simulink model "LQR_lpfnoise"  (R2022a)
settings: Solver=VariableStepAuto  StartTime=0.0  StopTime=25  RelTol=1e-3
values from neighbouring files (symbols this model uses):
  A = double(A)    [LQR.m]
  B = double(B)    [LQR.m]
undefined symbols (not defined in the file or in its folder): K
libraries: simulink x1, cstblocks x1
settings Model: Creator=Shiva  LastModifiedBy=amogh

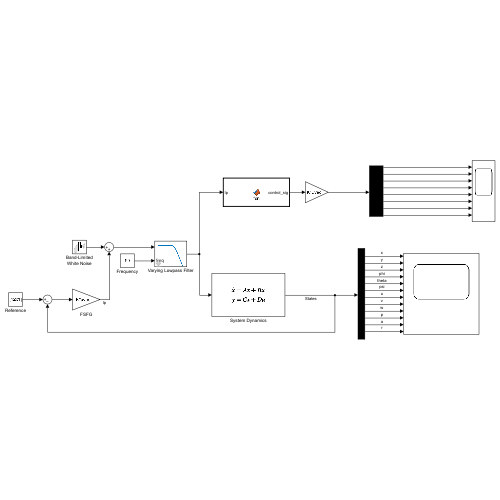
[thumbnail: Simulink's stored preview of the top-level diagram]
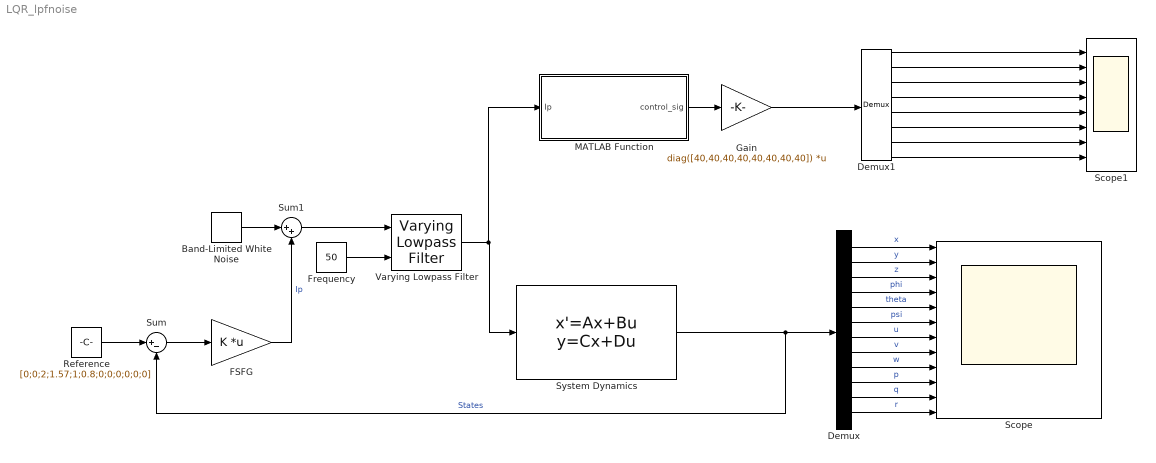
== system LQR_lpfnoise ==
  Band-Limited White Noise : simulink/Sources/Band-Limited White Noise  Cov=[0.1]  Ts=0.1  seed=[23341]
  Demux : Demux  Outputs=12
  Demux1 : Demux  Outputs=8
  FSFG : Gain  Gain=K  Multiplication=Matrix(K*u) (u vector)
  Frequency : Constant  Value=50
  Gain : Gain  Gain=diag([40,40,40,40,40,40,40,40])  Multiplication=Matrix(K*u) (u vector)
  MATLAB Function : MATLAB Function  TreatAsAtomicUnit=on
  Reference : Constant  Value=[0;0;2;1.57;1;0.8;0;0;0;0;0;0]  SampleTime=-1
  Scope : Scope  NumInputPorts=12
  Scope1 : Scope  NumInputPorts=8
  Sum : Sum  Inputs=|+-
  Sum1 : Sum  Inputs=|++
  System Dynamics : StateSpace  A=A  B=B  C=eye(12)  D=zeros(12,6)  InitialCondition=zeros(12,1)  ParameterTunability=Optimized
  Varying Lowpass Filter : cstblocks/Linear Parameter Varying/Varying Lowpass Filter  N=1
  wires:
  Reference/1 -> Sum/1
  System Dynamics/1 -> Sum/2, Demux/1  "States"
  Sum/1 -> FSFG/1
  Demux/1 -> Scope/1  "x"
  Demux/2 -> Scope/2  "y"
  Demux/3 -> Scope/3  "z"
  Demux/4 -> Scope/4  "phi"
  Demux/5 -> Scope/5  "theta"
  Demux/6 -> Scope/6  "psi"
  Demux/7 -> Scope/7  "u"
  Demux/8 -> Scope/8  "v"
  Demux/9 -> Scope/9  "w"
  Demux/10 -> Scope/10  "p"
  Demux/11 -> Scope/11  "q"
  Demux/12 -> Scope/12  "r"
  Demux1/1 -> Scope1/1
  Demux1/2 -> Scope1/2
  Demux1/3 -> Scope1/3
  Demux1/4 -> Scope1/4
  Demux1/5 -> Scope1/5
  Demux1/6 -> Scope1/6
  Demux1/7 -> Scope1/7
  Demux1/8 -> Scope1/8
  MATLAB Function/1(control_sig) -> Gain/1
  Gain/1 -> Demux1/1
  FSFG/1 -> Sum1/2  "Ip"
  Frequency/1 -> Varying Lowpass Filter/2
  Band-Limited White Noise/1 -> Sum1/1
  Sum1/1 -> Varying Lowpass Filter/1
  Varying Lowpass Filter/1 -> MATLAB Function/1(Ip), System Dynamics/1

== matlab function LQR_lpfnoise/MATLAB Function ==
  data: Ip input; control_sig output
function control_sig = fcn(Ip)
T=[0.707,0.707,-0.707,-0.707,0,0,0,0;
   -0.707,0.707,-0.707,0.707,0,0,0,0;
   0,0,0,0,-1,1,1,-1;
   0.06,-0.06,0.06,-0.06,-0.218,-0.218,0.218,0.218;
   0.06,0.06,-0.06,-0.06,0.120,-0.120,0.120,-0.120;
   -0.1888,0.1888,0.1888,-0.1888,0,0,0,0];

K=diag([40,40,40,40,40,40,40,40]);

T_star=(T.')*inv(T*(T.'));

control_sig=inv(K)*T_star*Ip;
